simulink model "plant"  (R2021b)
settings: Solver=VariableStepAuto  StartTime=0  StopTime=3000  RelTol=1e-3  AbsTol=1e-3
PreLoadFcn:
  | % Setup model parameters
  |                 % Sample time
  |                 Ts = 0.1;
  |                 % Simulation stop time ("TimeOut")
  |                 stop_time = 8000;
  |                 % Temperature
  |                 T_init = 20 + 273.1755;
  |                 T_final = 294.1755;
  |                 T_env = 20 + 273.15; %#ok<*NASGU>
  |                 % Heater
  |                 u_volts_heater_init = 0; % volts
  |                 % Pressure
  |                 p_init = 101.325; % kPa
  |                 p_env = 101.325; % kPa
  |                 % Relative humidity and steam
  |                 phi_init = 0.4987;
  |                 phi_final = 0.6;
  |                 phi_env = 0.1;
  |                 u_steam_init = 0;
  |                 T_steam = 130 + 273.15;
  |                 % Volumetric flow rate
  |                 u_volts_fan_init = 1;
  |                 flow_init = 5.8e-3;
  |                 flow_final = 0.18;
  |                 % Smooth ramp input parameters
  |                 smooth_step_heater = make_smooth_step(0, T_init, T_final, Ts, stop_time, 'T_g');
  |                 smooth_step_steam = make_smooth_step(0, phi_init, phi_final, Ts, stop_time, 'phi');
  |                 smooth_step_fan = make_smooth_step(0, flow_init, flow_final, Ts, stop_time, 'flow');
  |                 % Parameters to vary for linearization
  |                 % Pipes
  |                 pipe_length1 = 1; % meters
  |                 pipe_length2 = 1;
  |                 pipe_length3 = 1;
  |                 pipe_cross_sectional_area1 = pi*(2*2.54/2)^2; % cm^2
  |                 pipe_cross_sectional_area2 = pi*(2*2.54/2)^2;
  |                 pipe_cross_sectional_area3 = pi*(2*2.54/2)^2;
  |                 pipe_hydraulic_diameter1 = 2*2.54; %cm
  |                 pipe_hydraulic_diameter2 = 2*2.54; %cm
  |                 pipe_hydraulic_diameter3 = 2*2.54; %cm
  |                 % Thermal masses
  |                 thermal_mass1 = 1; % kg
  |                 thermal_mass2 = 1; % kg
  |                 thermal_mass3 = 1; % kg
  |                 thermal_mass4 = 1; % kg
  |                 thermal_mass5 = 1; % kg
  |                 specific_heat1 = 447; % J/(K*kg)
  |                 specific_heat2 = 447; % J/(K*kg)
  |                 specific_heat3 = 447; % J/(K*kg)
  |                 specific_heat4 = 447; % J/(K*kg)
  |                 specific_heat5 = 447; % J/(K*kg)
undefined symbols (not defined in the file or in its folder): c_volts_to_K
libraries: fl_lib x43, nesl_utility x20, SimscapeFluids_lib x1
(part 2 of 2)

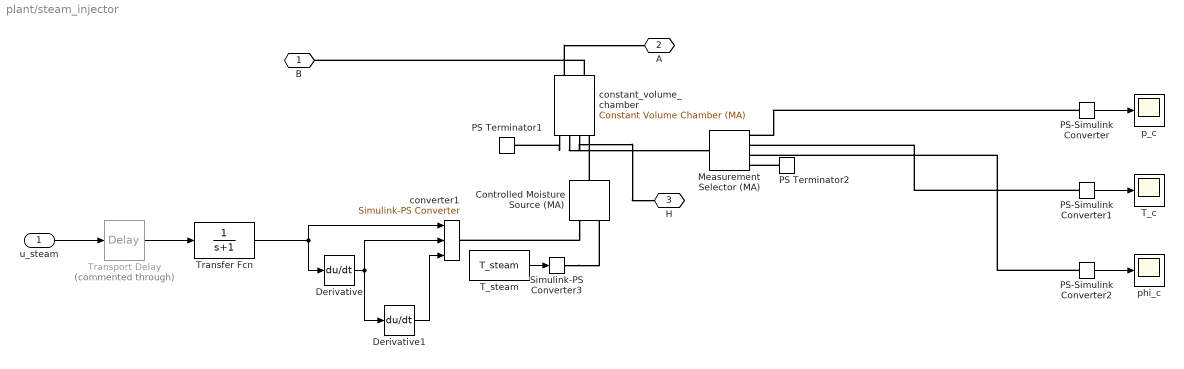
== system plant/steam_injector ==
  u_steam : Inport
  Controlled Moisture Source (MA) : fl_lib/Moist Air/Sources/Moisture & Trace Gas Sources/Controlled Moisture Source (MA)  moisture_source_spec=foundation.enum.moisture_source_spec.vapor  Phi_S_specify=off  Phi_S_priority=None  Phi_S=0 kW  Phi_S_nominal_specify=off  Phi_S_nominal_unit=kW  Phi_S_nominal_value=1  mdot_w_S_specify=off  mdot_w_S_priority=None  mdot_w_S=0 kg/s  mdot_w_S_nominal_specify=off  mdot_w_S_nominal_unit=kg/s  mdot_w_S_nominal_value=1
      settings: SourceProductBaseCode=SS  InternalSimscapePortConfiguration="{\"Bottom\":[],\"Left\":[{\"id\":\"S\",\"label\":\"S\",\"type\":\"foundation.moist_air.moist_air_source\"}],\"Right\":[{\"id\":\"M\",\"label\":\"M\",\"type\":\"input\"},{\"id\":\"T\",\"label\":\"T\",\"type\":\"input\"}],\"Top\":[]}"
  Derivative : Derivative
  Derivative1 : Derivative
  Measurement Selector (MA) : fl_lib/Moist Air/Sensors/Measurement Selector (MA)  moisture_spec=foundation.enum.moisture_spec.relative_humidity  trace_gas_spec=foundation.enum.trace_gas_spec.mass_fraction
      settings: SourceProductBaseCode=SS
  PS Terminator1 : fl_lib/Physical Signals/Sinks/PS Terminator
  PS Terminator2 : fl_lib/Physical Signals/Sinks/PS Terminator
  PS-Simulink Converter : nesl_utility/PS-Simulink Converter  PhysicalDomain=network_engine_domain  SubClassName=ps_output  LeftPortType=input  RightPortType=output  PseudoPeriodic=off  Frequencies=[]  Unit=kPa  AffineConversion=off
      settings: SourceProductBaseCode=PW,SS
  PS-Simulink Converter1 : nesl_utility/PS-Simulink Converter  PhysicalDomain=network_engine_domain  SubClassName=ps_output  LeftPortType=input  RightPortType=output  PseudoPeriodic=off  Frequencies=[]  Unit=K  AffineConversion=on
      settings: SourceProductBaseCode=PW,SS
  PS-Simulink Converter2 : nesl_utility/PS-Simulink Converter  PhysicalDomain=network_engine_domain  SubClassName=ps_output  LeftPortType=input  RightPortType=output  PseudoPeriodic=off  Frequencies=[]  Unit=1  AffineConversion=off
      settings: SourceProductBaseCode=PW,SS
  Simulink-PS Converter3 : nesl_utility/Simulink-PS Converter  PhysicalDomain=network_engine_domain  SubClassName=ps_input  LeftPortType=input  RightPortType=output  PseudoPeriodic=off  Frequencies=[]  NoiseDistribution=none  NoiseParameters=[]  Unit=K  AffineConversion=on  FilteringAndDerivatives=zero  SimscapeFilterOrder=1  InputFilterTimeConstant=0.001  UdotUserProvided=0
      settings: SourceProductBaseCode=PW,SS
  T_c : Scope
  T_steam : Constant  Value=T_steam
  Transfer Fcn : TransferFcn  Denominator=[1 1]
  Transport Delay : TransportDelay  Commented=through  BufferSize=1024000
  constant_volume_chamber : fl_lib/Moist Air/Elements/Constant Volume Chamber (MA)  volume=0.25 m^3  num_ports=foundation.enum.num_ports.two  area_A=pi*2^2 in^2  area_B=pi*2^2 in^2  area_C=pi*(2*2.54/2)^2 cm^2  area_D=0.01 m^2  RH_ws=1  time_constant=1e-3 s  moisture_trace_gas_source=foundation.enum.moisture_trace_gas_source.controlled  moisture_source_spec=foundation.enum.moisture_source_spec.vapor  moisture_mass_flow=0 kg/s  moisture_temperature_spec=foundation.enum.temperature_spec.atmospheric  moisture_temperature=293.15 K  trace_gas_mass_flow=0 kg/s  trace_gas_temperature_spec=foundation.enum.temperature_spec.atmospheric  trace_gas_temperature=293.15 K  p_I_specify=on  p_I_priority=None  p_I=p_init kPa  p_I_nominal_specify=off  p_I_nominal_unit=MPa  p_I_nominal_value=1  T_I_specify=on  T_I_priority=None  T_I=T_init K  T_I_nominal_specify=off  T_I_nominal_unit=K  T_I_nominal_value=1  RH_I_specify=on  RH_I_priority=None  RH_I=phi_init  RH_I_nominal_specify=off  RH_I_nominal_unit=1  RH_I_nominal_value=1  x_w_I_specify=off  x_w_I_priority=None  x_w_I=0  x_w_I_nominal_specify=off  x_w_I_nominal_unit=1  x_w_I_nominal_value=1  y_w_I_specify=off  y_w_I_priority=None  y_w_I=0  y_w_I_nominal_specify=off  y_w_I_nominal_unit=1  y_w_I_nominal_value=1  HR_I_specify=off  HR_I_priority=None  HR_I=0  HR_I_nominal_specify=off  HR_I_nominal_unit=1  HR_I_nominal_value=1  x_g_I_specify=off  x_g_I_priority=None  x_g_I=0  x_g_I_nominal_specify=off  x_g_I_nominal_unit=1  x_g_I_nominal_value=1  y_g_I_specify=off  y_g_I_priority=High  y_g_I=y_CO2_env  y_g_I_nominal_specify=off  y_g_I_nominal_unit=1  y_g_I_nominal_value=1
      settings: SourceProductBaseCode=SS  InternalSimscapePortConfiguration="{\"Bottom\":[],\"Left\":[{\"id\":\"A\",\"label\":\"A\",\"type\":\"foundation.moist_air.moist_air\"},{\"id\":\"B\",\"label\":\"B\",\"type\":\"foundation.moist_air.moist_air\"}],\"Right\":[{\"id\":\"W\",\"label\":\"W\",\"type\":\"output\"},{\"id\":\"F\",\"label\":\"F\",\"type\":\"output\"},{\"id\":\"H\",\"label\":\"H\",\"type\":\"foundation.thermal.thermal\"},{\"id\":\"S\",\"label\":\"S\",\"type\":\"foundation.moist_air.moist_air_source\"}],\"Top\":[]}"
  converter1 : nesl_utility/Simulink-PS Converter  PhysicalDomain=network_engine_domain  SubClassName=ps_input  LeftPortType=input  RightPortType=output  PseudoPeriodic=off  Frequencies=[]  NoiseDistribution=none  NoiseParameters=[]  Unit=kg/s  AffineConversion=off  FilteringAndDerivatives=provide  SimscapeFilterOrder=1  InputFilterTimeConstant=0.001  UdotUserProvided=2
      settings: SourceProductBaseCode=PW,SS
  p_c : Scope
  phi_c : Scope
  B : PMIOPort  Side=Left
  A : PMIOPort  Port=2  Side=Right
  H : PMIOPort  Port=3  Side=Right
  wires:
  T_steam/1 -> Simulink-PS Converter3/1
  u_steam/1 -> Transport Delay/1
  PS-Simulink Converter2/1 -> phi_c/1
  PS-Simulink Converter1/1 -> T_c/1
  PS-Simulink Converter/1 -> p_c/1
  Transfer Fcn/1 -> Derivative/1, converter1/1
  Derivative/1 -> Derivative1/1, converter1/2
  Derivative1/1 -> converter1/3
  Transport Delay/1 -> Transfer Fcn/1
  connections:
  constant_volume_chamber/RConn1 -- PS Terminator1/LConn1
  constant_volume_chamber/LConn1 -- A/RConn1
  Controlled Moisture Source (MA)/LConn1 -- constant_volume_chamber/RConn4
  constant_volume_chamber/RConn2 -- Measurement Selector (MA)/LConn1
  Simulink-PS Converter3/RConn1 -- Controlled Moisture Source (MA)/RConn2
  constant_volume_chamber/RConn3 -- H/RConn1
  Controlled Moisture Source (MA)/RConn1 -- converter1/RConn1
  constant_volume_chamber/LConn2 -- B/RConn1
  PS-Simulink Converter/LConn1 -- Measurement Selector (MA)/RConn1
  PS-Simulink Converter2/LConn1 -- Measurement Selector (MA)/RConn3
  PS-Simulink Converter1/LConn1 -- Measurement Selector (MA)/RConn2
  PS Terminator2/LConn1 -- Measurement Selector (MA)/RConn4
